simulink model "Attitude_Estimation"  (R2026a)
settings: Solver=VariableStepAuto
model workspace (MAT data in the model file):
  P_wahba = Simulink.Parameter
  P_wahba.Complexity = 'real'
  P_wahba.Dimensions = [0 0]
  P_wahba.DataType = 'auto'
  q_opt = 0
values from neighbouring files (symbols this model uses):
  P_wahba = reshape(P_wahba, 3, 3)    [matrice_P_0.m]    (also in solve_wahba_q_method.m = sigmatot^2 * inv(Info_matrix))
undefined symbols (not defined in the file or in its folder): IGRF
libraries: vrlib x1
settings Model: Creator=aless  LastModifiedBy=aless

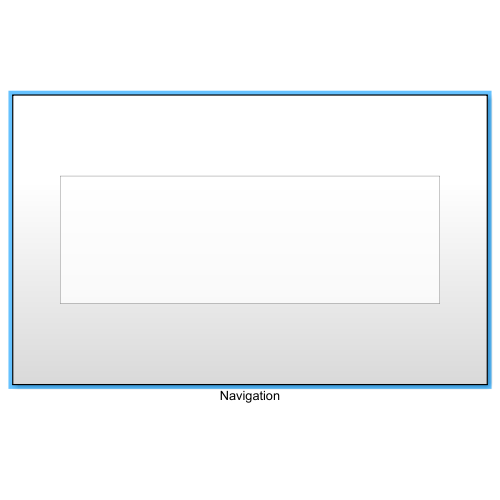
[thumbnail: Simulink's stored preview of the top-level diagram]
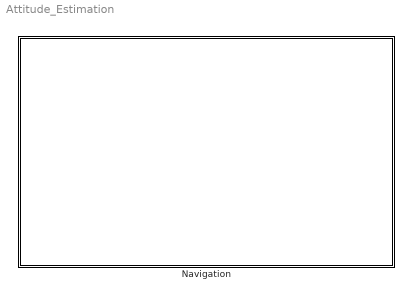
== system Attitude_Estimation ==
  Navigation : Subsystem

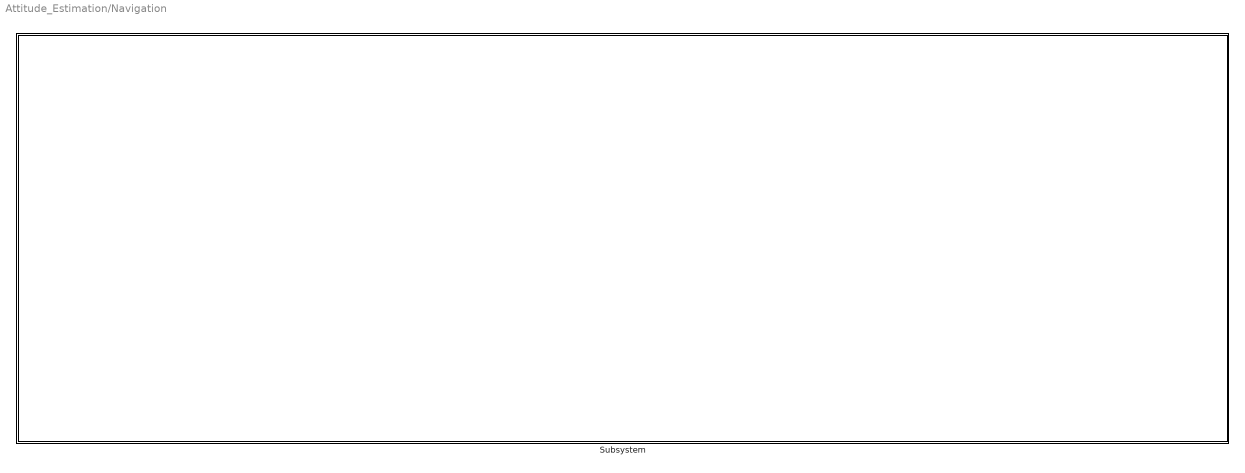
== system Attitude_Estimation/Navigation ==
  Subsystem : Subsystem

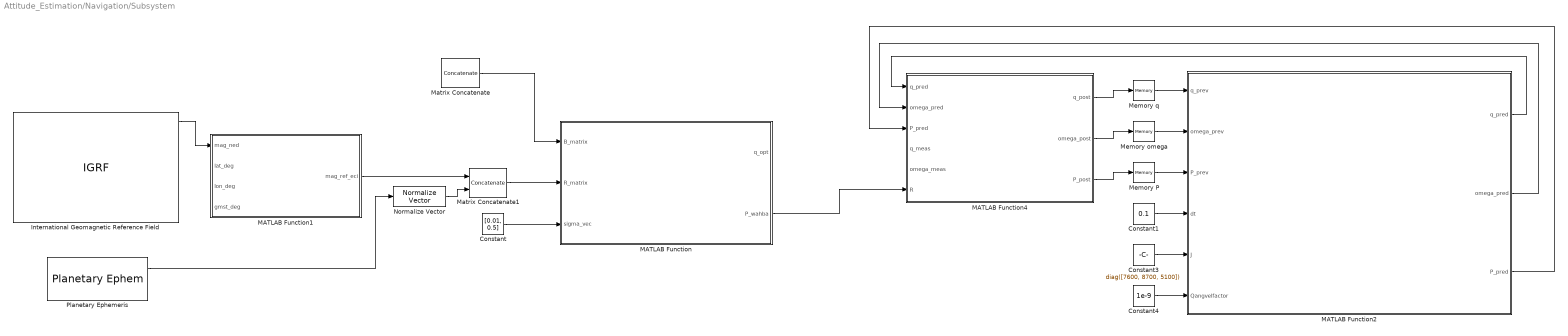
== system Attitude_Estimation/Navigation/Subsystem ==
  Constant : Constant  Value=[0.01, 0.5]
  Constant1 : Constant  Value=0.1
  Constant3 : Constant  Value=diag([7600, 8700, 5100])
  Constant4 : Constant  Value=1e-9
  International Geomagnetic Reference Field : IGRF  generation=IGRF-13  month=January  day=1
      settings: AttributesFormatString=%<generation>
  MATLAB Function : MATLAB Function  TreatAsAtomicUnit=on
  MATLAB Function1 : MATLAB Function  TreatAsAtomicUnit=on
  MATLAB Function2 : MATLAB Function  TreatAsAtomicUnit=on
  MATLAB Function4 : MATLAB Function  TreatAsAtomicUnit=on
  Matrix Concatenate : Concatenate  Mode=Multidimensional array  ConcatenateDimension=2
  Matrix Concatenate1 : Concatenate  Mode=Multidimensional array  ConcatenateDimension=2
  Memory P : Memory  InitialCondition=P_wahba
  Memory omega : Memory  InitialCondition=[0.1; 0.1; 0.1]
  Memory q : Memory  InitialCondition=q_opt
  Normalize Vector : vrlib/Utilities/Normalize Vector  maxzero=0
  Planetary Ephemeris : PlanetaryEphem  target=Sun
  wires:
  Matrix Concatenate1/1 -> MATLAB Function/2(R_matrix)
  Matrix Concatenate/1 -> MATLAB Function/1(B_matrix)
  MATLAB Function1/1(mag_ref_eci) -> Matrix Concatenate1/1
  Planetary Ephemeris/1 -> Normalize Vector/1
  Constant/1 -> MATLAB Function/3(sigma_vec)
  Normalize Vector/1 -> Matrix Concatenate1/2
  International Geomagnetic Reference Field/1 -> MATLAB Function1/1(mag_ned)
  Constant1/1 -> MATLAB Function2/4(dt)
  Constant3/1 -> MATLAB Function2/5(J)
  Constant4/1 -> MATLAB Function2/6(Qangvelfactor)
  Memory P/1 -> MATLAB Function2/3(P_prev)
  Memory omega/1 -> MATLAB Function2/2(omega_prev)
  Memory q/1 -> MATLAB Function2/1(q_prev)
  MATLAB Function4/1(q_post) -> Memory q/1
  MATLAB Function2/1(q_pred) -> MATLAB Function4/1(q_pred)
  MATLAB Function2/2(omega_pred) -> MATLAB Function4/2(omega_pred)
  MATLAB Function2/3(P_pred) -> MATLAB Function4/3(P_pred)
  MATLAB Function/2(P_wahba) -> MATLAB Function4/6(R)
  MATLAB Function4/2(omega_post) -> Memory omega/1
  MATLAB Function4/3(P_post) -> Memory P/1

== matlab function Attitude_Estimation/Navigation/Subsystem/MATLAB Function1 ==
  data: mag_ned input; mag_ref_eci output; lat_deg input; lon_deg input; gmst_deg input
function mag_ref_eci = transform_ned_to_eci(mag_ned, lat_deg, lon_deg, gmst_deg)
% TRASFORMAZIONE CAMPO MAGNETICO: NED -> ECEF -> ECI
% INPUTS:
%   mag_ned  : Collegare DIRETTAMENTE al PRIMO OUTPUT del blocco IGRF 13
%   lat_deg  : Latitudine geodetica istantanea [gradi] (dalla propagazione orbitale)
%   lon_deg  : Longitudine geodetica istantanea [gradi] (dalla propagazione orbitale)
%   gmst_deg : Greenwich Mean Sidereal Time [gradi] (da Julian Date to GMST block)
% OUTPUT:
%   mag_ref_eci: Vettore direzione 3x1 normalizzato in ECI (per Wahba R_matrix)

% --- SICUREZZA INGRESSO (Robusta per Simulink) ---
% Forza il vettore in ingresso a essere una colonna 3x1,
% indipendentemente se Simulink lo invia come riga (1x3) o colonna (3x1).
mag_ned = mag_ned(:); 

% Conversione in radianti per le funzioni trigonometriche
lat = deg2rad(lat_deg);
lon = deg2rad(lon_deg);
gmst = deg2rad(gmst_deg);

% --- 1. MATRICE DI ROTAZIONE: NED -> ECEF ---
% Basata sulle coordinate geodetiche del satellite
R_ned_to_ecef = [ -sin(lat)*cos(lon), -sin(lon), -cos(lat)*cos(lon);
    -sin(lat)*sin(lon),  cos(lon), -cos(lat)*sin(lon);
    cos(lat),           0,        -sin(lat) ];

% --- 2. MATRICE DI ROTAZIONE: ECEF -> ECI ---
% Basata sulla rotazione terrestre istantanea (GMST)
R_ecef_to_eci = [ cos(gmst), -sin(gmst), 0;
    sin(gmst),  cos(gmst), 0;
    0,          0,         1 ];

% --- 3. TRASFORMAZIONE COMPLETA ---
% v_eci = R(ECEF->ECI) * R(NED->ECEF) * v_ned
mag_eci_unnorm = R_ecef_to_eci * R_ned_to_ecef * mag_ned;

% --- 4. NORMALIZZAZIONE (Essenziale per Wahba) ---
% Eliminiamo l'intensità (nT) e teniamo solo la direzione
norm_val = norm(mag_eci_unnorm);
if norm_val < 1e-9 % Protezione contro divisione per zero
    mag_ref_eci = [0; 0; 0]; 
else
    mag_ref_eci = mag_eci_unnorm / norm_val;
end
end

== matlab function Attitude_Estimation/Navigation/Subsystem/MATLAB Function ==
  data: B_matrix input; q_opt output; R_matrix input; sigma_vec input; P_wahba output
function [q_opt, P_wahba] = solve_wahba_q_method(B_matrix, R_matrix, sigma_vec)
% Risolutore Wahba Q-method (scalar-last quaternion)

% INPUT:
%   B_matrix : 3xN vettori misurati in body frame (colonne, non normalizzati)
%   R_matrix : 3xN vettori di riferimento in reference frame (colonne)
%   sigma_vec: 1xN deviazioni standard angolari delle misure [gradi],
%   ovvero quanto sono precisi i sensori

% OUTPUT:
%   q_opt   : quaternione ottimale [q1 q2 q3 q4], scalar-last
%   P_wahba : covarianza 3x3 dell'errore in dtheta [rad^2]

if nargin == 0
    % --- BLOCCO DI AUTODIAGNOSTICA / UNIT TESTING ---
    % Best practice: permette di runnare lo script a vuoto per verificare che funzioni.
    % Test di default coerente col progetto ADCS (2 sensori, es. Sun Sensor e Magnetometro)
    B_matrix = [0; -1; 0];           % es. sun sensor body
    B_matrix(:,2) = [0.6; 0; 0.8];   % es. magnetometro body
    R_matrix = [0; -1; 0];
    R_matrix(:,2) = [0.6; 0; 0.8];
    sigma_vec = [0.01, 0.5];         % gradi: star tracker, magnetometro
    [q_opt, P_wahba] = solve_wahba_q_method(B_matrix, R_matrix, sigma_vec);
    disp('q_opt:'); disp(q_opt');
    disp('P_wahba sqrt diag (deg):');
    disp(sqrt(diag(P_wahba))' * 180/pi);
    return
end

N = size(B_matrix, 2);
sigma_rad = deg2rad(sigma_vec);   % converti in radianti

% --- CALCOLO PESI NORMALIZZATI ---
% L'algoritmo deve fidarsi di più dei sensori precisi (es. Star Tracker).
% sigmatot rappresenta la deviazione standard equivalente globale del set.
sigmatot = 1 / sqrt(sum(1 ./ sigma_rad.^2));
a = sigmatot^2 ./ sigma_rad.^2;   % Pesi normalizzati: sum(a) = 1

% --- Attitude Profile Matrix B ---
Bmat = zeros(3,3);
z    = zeros(3,1);
for i = 1:N
    % Normalizzazione di sicurezza per evitare errori da sensori/modelli
    b_i = B_matrix(:,i) / norm(B_matrix(:,i));
    r_i = R_matrix(:,i) / norm(R_matrix(:,i));
    % Bmat: Matrice 3x3 che condensa tutte le info direzionali pesate.
    Bmat = Bmat + a(i) * (b_i * r_i');
    % z: Vettore che cattura l'errore fisico di disallineamento incrociato.
    z    = z    + a(i) * cross(b_i, r_i);
end

% --- MATRICE DI DAVENPORT (K) ---
% Davenport trasforma il problema di minimizzazione di Wahba in un
% problema agli autovalori sui quaternioni.
S     = Bmat + Bmat';
sigma = trace(Bmat);
K = [ S - sigma*eye(3),  z ;
    z'              ,  sigma ]; % Struttura valida per convenzione SCALAR-LAST

% --- SOLUZIONE AGLI AUTOVALORI (IL Q-METHOD) ---
[V, D] = eig(K);
% Il quaternione che minimizza la loss function è l'autovettore
% corrispondente all'autovalore MASSIMO della matrice K.
[~, idx] = max(diag(D));
q_opt = V(:, idx);

% --- SANITY CHECK: AMBIGUITÀ EMISFERICA ---
% I quaternioni q e -q descrivono la stessa rotazione fisica.
% Forziamo la parte scalare positiva per evitare fastidiosi "salti di segno" 
% (unwinding) che manderebbero in instabilità la propagazione nel MEKF.
if q_opt(4) < 0
    q_opt = -q_opt;
end

% --- COVARIANZA IN dtheta [rad^2] (FISHER INFORMATION MATRIX) ---
% Generiamo il dato sul rumore della misura d'assetto da passare al Kalman Filter.
sum_weighted_outer = zeros(3,3);
for i = 1:N
    b_i = B_matrix(:,i) / norm(B_matrix(:,i));
    sum_weighted_outer = sum_weighted_outer + a(i) * (b_i * b_i');
end

% Info_matrix quantifica la bontà geometrica delle misurazioni attuali.
Info_matrix = eye(3) - sum_weighted_outer;

% --- CONTROLLO DI ROBUSTEZZA ---
% Se i vettori misurati sono paralleli (es. Sole e Campo Magnetico allineati), 
% si perde un grado di libertà e la matrice diventa quasi-singolare.
if rcond(Info_matrix) < 1e-12
    warning('Info_matrix quasi-singolare: configurazione geometrica degenere.');
    % Evita il crash di Simulink calcolando la pseudo-inversa (pinv)
    P_wahba = pinv(Info_matrix) * sigmatot^2;
else
    % Condizione operativa nominale
    P_wahba = sigmatot^2 * inv(Info_matrix);
end
end

== matlab function Attitude_Estimation/Navigation/Subsystem/MATLAB Function2 ==
  data: q_prev input; q_pred output; omega_prev input; P_prev input; dt input; J input; Qangvelfactor input; omega_pred output; P_pred output
function [q_pred, omega_pred, P_pred] = mekf_prediction_step(q_prev, omega_prev, P_prev, dt, J, Qangvelfactor)
% MEKF PREDICTION STEP - Propagazione stato e covarianza

% INPUT:
%   q_prev        : quaternione [4x1] al passo k-1, scalar-last [q1 q2 q3 q4]
%                   All'inizializzazione: q_prev = q_opt da solve_wahba_q_method
%   omega_prev    : velocita' angolare [3x1] al passo k-1 [rad/s]
%   P_prev        : covarianza [6x6] al passo k-1
%                   All'inizializzazione: assemblare come
%                     P_prev = [P_wahba, zeros(3,3); zeros(3,3), sigma_omega^2*eye(3)]
%                   con P_wahba da solve_wahba_q_method e
%                   sigma_omega = 2e-4 rad/s (Astrix 1090, datasheet)
%   dt            : passo di integrazione [s]
%   J             : matrice d'inerzia 3x3 [kg*m^2]
%                   Per il progetto: diag([7600, 8700, 5100])
%   Qangvelfactor : PSD del rumore angolare [rad^2/s^3], scalare
%                   Stima da Astrix 1090 ARW = 0.005 deg/sqrt(h):
%                   ARW_rad = 0.005/sqrt(3600)*pi/180 = 1.45e-6 rad/sqrt(s)
%                   Qangvelfactor = ARW_rad^2 = ~2.1e-12 rad^2/s^3
%                   In pratica nel progetto si usa 1e-9 (margine conservativo)
%
% OUTPUT:
%   q_pred     : quaternione propagato [4x1], scalar-last, rinormalizzato
%   omega_pred : velocita' angolare propagata [3x1] [rad/s]
%   P_pred     : covarianza propagata [6x6]

%% 1. PROPAGAZIONE QUATERNIONE
% Usa propagate_quaternion (funzione del progetto) che implementa
% l'integrazione della cinematica q_dot = (1/2)*Omega(omega)*q
q_pred = propagate_quaternion(q_prev, omega_prev, dt);
% propagate_quaternion include gia' la rinormalizzazione interna.

%% 2. PROPAGAZIONE VELOCITA' ANGOLARE (Equazioni di Eulero senza coppia esterna)
% omega_dot = J^{-1} * (-(omega x J*omega))
% La coppia esterna e' gestita nel correction step o come disturbance
% nel Q_proc, non nella predizione nominale.
skew_omega = [0,            -omega_prev(3),  omega_prev(2);
    omega_prev(3),  0,            -omega_prev(1);
    -omega_prev(2),  omega_prev(1),  0           ];

omega_dot  = inv(J) * (-(skew_omega * J * omega_prev));
omega_pred = omega_prev + omega_dot .* dt;

%% 3. JACOBIANO DEL PROCESSO F (6x6)
% Linearizzazione attorno allo stato corrente, coerente con JacobProcess
Jomega     = J * omega_prev;
skew_Jomega = [0,          -Jomega(3),  Jomega(2);
    Jomega(3),   0,         -Jomega(1);
    -Jomega(2),   Jomega(1),  0         ];

F = [-skew_omega,    0.5*eye(3);
    zeros(3,3),    inv(J)*(-skew_omega*J + skew_Jomega)];

%% 4. MATRICE DI TRANSIZIONE Phi (esponenziale di matrice)
% expm e' piu' accurata di eye(6)+F*dt per dt non trascurabili.
Phi = expm(F .* dt);

%% 5. Q DISCRETA (Metodo di Van Loan)
% G: matrice di ingresso del rumore - il rumore di processo agisce SOLO
% sulle 3 componenti di velocita' angolare (non sull'attitude direttamente).
G = [zeros(3,3); eye(3)];

% Van Loan: trasforma l'integrale della covarianza discreta in un esponenziale
% Qd = int_0^dt [Phi(tau)*G*q*G'*Phi(tau)'] dtau
M = [-F,                  G * Qangvelfactor * G';
    zeros(6),           F'                   ] .* dt;

E   = expm(M);
Phi_vl = E(7:12, 7:12)';     % recupera Phi dal blocco in basso a destra
Qd  = Phi_vl * E(1:6, 7:12); % covarianza discreta

%% 6. PROPAGAZIONE COVARIANZA
P_pred = Phi * P_prev * Phi' + Qd;

% Simmetrizzazione numerica (previene deriva per accumulo di errori float)
P_pred = (P_pred + P_pred') / 2;

end

== matlab function Attitude_Estimation/Navigation/Subsystem/MATLAB Function4 ==
  data: q_pred input; q_post output; omega_pred input; P_pred input; q_meas input; omega_meas input; R input; omega_post output; P_post output
function [q_post, omega_post, P_post] = mekf_correction_step(q_pred, omega_pred, P_pred, q_meas, omega_meas, R)

% =========================================================================
% MEKF CORRECTION STEP - Aggiornamento stato e covarianza
% =========================================================================

% INPUT:
%   q_pred     : quaternione predetto [4x1], scalar-last, da mekf_prediction_step
%   omega_pred : velocita' angolare predetta [3x1] [rad/s], da mekf_prediction_step
%   P_pred     : covarianza predetta [6x6], da mekf_prediction_step
%   q_meas     : quaternione misurato dallo Star Tracker [4x1], scalar-last
%                (ASTRO APS: accuratezza < 1 arcsec across boresight, 1-sigma)
%   omega_meas : velocita' angolare misurata dai giroscopi [3x1] [rad/s]
%                (Astrix 1090: ARW < 0.005 deg/sqrt(h), bias < 0.01 deg/h)
%   R          : matrice di covarianza delle misure [6x6]
%                Struttura:
%                  std_phidq    = 1 deg (Star Tracker, 1-sigma)
%                  Rattitude    = (std_phidq*pi/180)^2 / 12 * eye(3)
%                  Rangvel      = Sigma_omegameas^2 * eye(3)
%                  R = blkdiag(Rattitude, Rangvel)
%
% OUTPUT:
%   q_post     : quaternione corretto e rinormalizzato [4x1], scalar-last
%   omega_post : velocita' angolare corretta [3x1] [rad/s]
%   P_post     : covarianza aggiornata [6x6], simmetrica e definita positiva

% =========================================================================
% 1. INNOVAZIONE (RESIDUO)
% =========================================================================

% --- Innovazione di assetto ---
% Calcola il quaternione errore tra misura e predizione:
%   dq = q_meas * q_pred^{-1}
% Per un quaternione unitario: q^{-1} = q* = [-qv; qs]
q_pred_conj = [-q_pred(1:3); q_pred(4)];            % coniugato = inverso
dq_inn = q_product(q_meas, q_pred_conj);             % quaternione errore

% Correzione emisferica: impone dq_s >= 0 per evitare salti di segno
% nell'innovazione che causerebbero instabilita' durante la convergenza.
if dq_inn(4) < 0
    dq_inn = -dq_inn;
end

% Innovazione in termini di vettore di Gibbs: dg = dq_v / dq_s
% (approssimazione: dg ≈ dθ/2 per piccoli angoli)
% La distinzione e' importante durante la convergenza iniziale.
delta_g_inn = dq_inn(1:3) ./ dq_inn(4);             % vettore di Gibbs [3x1]

% --- Innovazione di velocita' angolare ---
delta_omega_inn = omega_meas - omega_pred;           % residuo omega [3x1]

% --- Vettore di innovazione completo ---
innovation = [delta_g_inn; delta_omega_inn];         % [6x1]

% =========================================================================
% 2. GUADAGNO DI KALMAN
% =========================================================================
% H = I(6x6): il modello di misura e' diretto (stato = misura).
H = eye(6);

% Matrice di innovazione S = H*P*H' + R = P_pred + R (poiche' H=I)
S = P_pred + R;                                      % [6x6]

% Guadagno ottimale: K = P * H' * S^{-1} = P_pred * S^{-1}
K = P_pred * (S \ eye(6));                           % [6x6], equivale a P/S

% =========================================================================
% 3. AGGIORNAMENTO DELLO STATO D'ERRORE
% =========================================================================
% Correzione nello spazio degli errori: delta_x = K * innovation
delta_x = K * innovation;                            % [6x1]

dg_up  = delta_x(1:3);   % errore d'assetto stimato (Gibbs vector) [3x1]
dw_up  = delta_x(4:6);   % errore di velocita' angolare stimato [3x1]

% =========================================================================
% 4. RESET (iniezione dell'errore nello stato globale)
% =========================================================================

% --- Aggiornamento moltiplicativo del quaternione ---
% Converte il vettore di Gibbs dg in quaternione d'errore normalizzato.
% Formula: dq_k = [dg; 1] / sqrt(1 + ||dg||^2)
dq_up = [dg_up; 1] / sqrt(1 + dg_up' * dg_up);     % quaternione d'errore [4x1]

% Composizione moltiplicativa: q_post = dq_up * q_pred
q_post = q_product(dq_up, q_pred);
q_post = q_post / norm(q_post);                      % rinormalizzazione di sicurezza

% --- Aggiornamento additivo della velocita' angolare ---
omega_post = omega_pred + dw_up;                     % [3x1], rad/s

% =========================================================================
% 5. AGGIORNAMENTO DELLA COVARIANZA
% =========================================================================
% Forma di Joseph: P = (I-KH)*P*(I-KH)' + K*R*K'
% Garantisce la definita positività di P anche con errori numerici,
% necessario per #codegen su hardware embedded (GR740 OBC).
% La forma standard (I-KH)*P e' numericamente instabile se K non e' ottimale.
IKH   = eye(6) - K * H;                             % [6x6]
P_post = IKH * P_pred * IKH' + K * R * K';          % forma di Joseph

% Simmetrizzazione finale per robustezza numerica
P_post = (P_post + P_post') / 2;

end
